simulink model "MCU_regionalPolePlacementLMI_SAME54_MCLV2"  (R2023b)
settings: Solver=FixedStepDiscrete  StartTime=0.0  StopTime=10.0  FixedStep=5e-5  RelTol=1e-3  EnableMultiTasking=on
InitFcn:
  | % DC Voltage
  | VDC = 24;
  | 
  | % Intersective PMW
  | Vmax = VDC/2;
  | Imax = 4;
  | 
  | Ts = 1e-4;
  | 
  | % pole paires
  | p = 4;
  | 
  | % QEI
  | lines = 4*1000;
  | eleclines = lines/p;
  | inveleclines = 1/eleclines
  | gainQEIspeed = 2*pi/Ts/lines
  | 
  | model.R = 0.656;         % Ohm
  | model.L = 0.35e-3;       % H
  | model.Phif = 6.6e-3;     % Wb
  | model.p = 4;
  | model.F = 1.e-05;
  | model.J = 1e-05;
  | disp(model);
  | 
  | % State space representation of the motor model
  | 
  | A = [-model.R/model.L -model.p*model.Phif ; 3*model.p*model.Phif/(2*model.J) -model.F/model.J ];
  | B = [1/model.L;0];
  | C = [0 1];
  | n=size(A,1);
  | % Augmented model with integral action
  | 
  | n=size(A,1); mx=size(B,2);
  | 
  | warning('off')
  | A = [A zeros(n,1);-C 0] ;
  | Bu=[B;0];Bw=[eye(3)];Duz=[1];Cz=[0 0 0];
  | 
  | n= 3;
  | m = 1;
  | 
  | %%% LIST OF UKNOWNS (lambda is the first, always included)
  | Nunk=uint16(2);
  | nunk = 1;
  | %UNK=cell(Nunk,1);
  | UNK = struct(...
  |     ...%'lab',{'X','Y'},...
  |     'col',{uint16(n),uint16(n)},...
  |     'row',{uint16(n),uint16(m)},...
  |     'sym',{uint16(1),uint16(0)},...
  |     'start',{uint16(0),uint16(0)},...
  |     'siz',{uint16(n*(n+1)/2),uint16(n*m)},...
  |     'X',{single(zeros(n,n,n*(n+1)/2)),single(zeros(m,n,n*m))},...
  |     'ste',{single(zeros(n,n)),single(zeros(m,n))},...
  |     'end',{uint16(nunk),uint16(nunk)}...
  |    );
  | 
  | 
  | ... (+100 lines)
undefined symbols (not defined in the file or in its folder): ADC0, AIN0, AIN6, B27, DiscIntNeverNeededParam, NumBits1, NumBits2, PA02, PA03, PA06, PA08, PA09, PA10, PA11, PA12, PA13, PA16, PA17, PA18, pad0, pad1, pad2, pad3, PB08, PC16, PC17, PC18, Pin, SAME54P20A, TQFP128, VREFA, wo0, wo1, wo2, wo4, wo5, wo6
libraries: simulink x20, MCHP_Blockset x12, dspfdesign x1
(part 2 of 3)

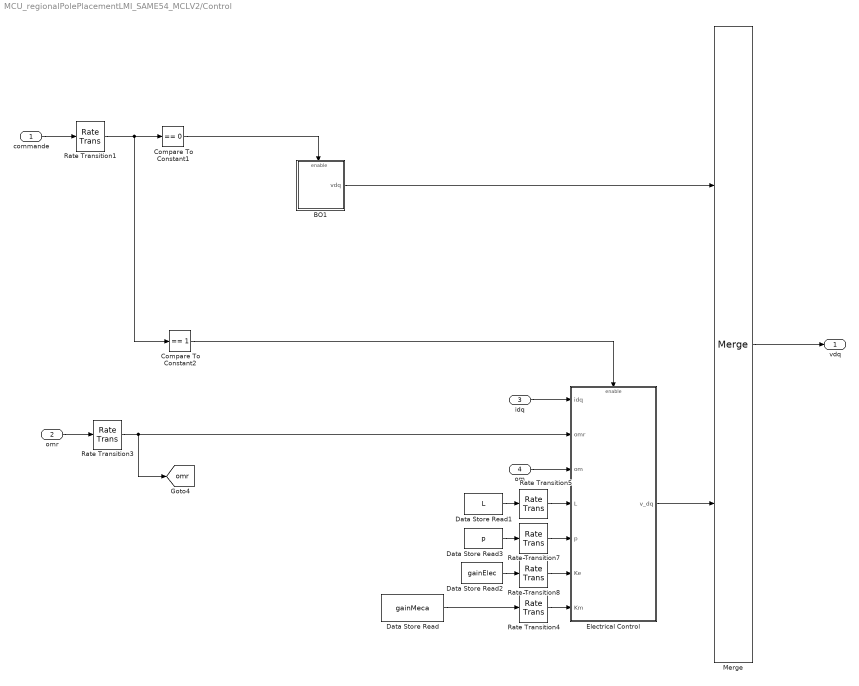
== system MCU_regionalPolePlacementLMI_SAME54_MCLV2/Control ==
  commande : Inport
  omr : Inport  Port=2
  idq : Inport  Port=3
  om : Inport  Port=4
  BO1 : Subsystem
  Compare To Constant1 : simulink/Logic and Bit Operations/Compare To Constant  relop===  const=0  OutDataTypeStr=boolean
  Compare To Constant2 : simulink/Logic and Bit Operations/Compare To Constant  relop===  const=1  OutDataTypeStr=boolean
  Data Store Read : DataStoreRead  DataStoreName=gainMeca  IndexOptions=Index vector (dialog)  Indices=1  OutputSizes=1
  Data Store Read1 : DataStoreRead  DataStoreName=L  SampleTime=1  IndexOptions=Index vector (dialog)  Indices=1  OutputSizes=1
  Data Store Read2 : DataStoreRead  DataStoreName=gainElec  IndexOptions=Index vector (dialog)  Indices=1  OutputSizes=1
  Data Store Read3 : DataStoreRead  DataStoreName=p  SampleTime=1  IndexOptions=Index vector (dialog)  Indices=1  OutputSizes=1
  Electrical Control : Subsystem
  Merge : Merge
  Rate Transition{1,3..5,7..8} (6 alike) : RateTransition
  vdq : Outport  VectorParamsAs1DForOutWhenUnconnected=off
  tag scope: omr=global
  wires:
  idq/1 -> Electrical Control/1(idq)
  Rate Transition1/1 -> Compare To Constant1/1, Compare To Constant2/1
  Compare To Constant1/1 -> BO1/Enable
  commande/1 -> Rate Transition1/1
  Merge/1 -> vdq/1
  Compare To Constant2/1 -> Electrical Control/Enable
  BO1/1(vdq) -> Merge/1
  Rate Transition3/1 -> [omr], Electrical Control/2(omr)
  Data Store Read3/1 -> Rate Transition7/1
  Data Store Read1/1 -> Rate Transition5/1
  Data Store Read2/1 -> Rate Transition8/1
  Electrical Control/1(v_dq) -> Merge/2
  Rate Transition5/1 -> Electrical Control/4(L)
  Rate Transition7/1 -> Electrical Control/5(p)
  Rate Transition8/1 -> Electrical Control/6(Ke)
  om/1 -> Electrical Control/3(om)
  omr/1 -> Rate Transition3/1
  Data Store Read/1 -> Rate Transition4/1
  Rate Transition4/1 -> Electrical Control/7(Km)

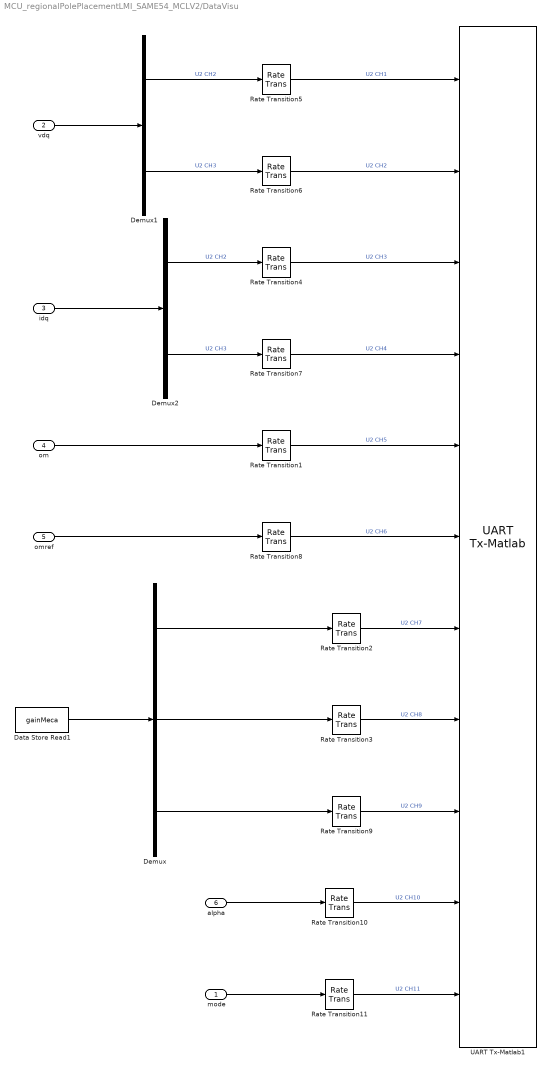
== system MCU_regionalPolePlacementLMI_SAME54_MCLV2/DataVisu ==
  mode : Inport
  vdq : Inport  Port=2
  idq : Inport  Port=3
  om : Inport  Port=4
  omref : Inport  Port=5
  alpha : Inport  Port=6
  Data Store Read1 : DataStoreRead  DataStoreName=gainMeca  IndexOptions=Index vector (dialog)  Indices=1  OutputSizes=1
  Demux : Demux  Outputs=3
  Demux1 : Demux  Outputs=2
  Demux2 : Demux  Outputs=2
  Rate Transition{1..9} (9 alike) : RateTransition
  Rate Transition10 : RateTransition  Integrity=off
  Rate Transition11 : RateTransition  Integrity=off
  UART Tx-Matlab1 : MCHP_Blockset/BUS UART/UART Tx-Matlab  UART_REF=2  CHANNELS=[1:11]  AllOrNothing=off  SampleTime=0.001  MCHP_MASTERLINK=MCU_regionalPolePlacementLMI_SAME54_MCLV2/Microchip Master  MCHP_COMPILED_INFO="CompiledSampleTime= [0.0010000000000000000208   0 ];CompiledInportDataTypes=[  1   1   1   1   1   1   1   1   1   1   5 ];CompiledInportDataWidth=[1  1  1  1  1  1  1  1  1  1  1];"
      settings: SourceProductName=MPLAB Device Blocks for Simulink
  wires:
  vdq/1 -> Demux1/1
  idq/1 -> Demux2/1
  omref/1 -> Rate Transition8/1
  Demux2/2 -> Rate Transition7/1  "U2 CH3"
  Demux2/1 -> Rate Transition4/1  "U2 CH2"
  Rate Transition5/1 -> UART Tx-Matlab1/1  "U2 CH1"
  Rate Transition8/1 -> UART Tx-Matlab1/6  "U2 CH6"
  Rate Transition1/1 -> UART Tx-Matlab1/5  "U2 CH5"
  Demux1/2 -> Rate Transition6/1  "U2 CH3"
  Rate Transition6/1 -> UART Tx-Matlab1/2  "U2 CH2"
  Rate Transition4/1 -> UART Tx-Matlab1/3  "U2 CH3"
  Demux1/1 -> Rate Transition5/1  "U2 CH2"
  om/1 -> Rate Transition1/1
  Rate Transition7/1 -> UART Tx-Matlab1/4  "U2 CH4"
  Rate Transition2/1 -> UART Tx-Matlab1/7  "U2 CH7"
  Rate Transition3/1 -> UART Tx-Matlab1/8  "U2 CH8"
  Rate Transition9/1 -> UART Tx-Matlab1/9  "U2 CH9"
  Demux/1 -> Rate Transition2/1
  Demux/2 -> Rate Transition3/1
  Demux/3 -> Rate Transition9/1
  Data Store Read1/1 -> Demux/1
  Rate Transition10/1 -> UART Tx-Matlab1/10  "U2 CH10"
  alpha/1 -> Rate Transition10/1
  mode/1 -> Rate Transition11/1
  Rate Transition11/1 -> UART Tx-Matlab1/11  "U2 CH11"

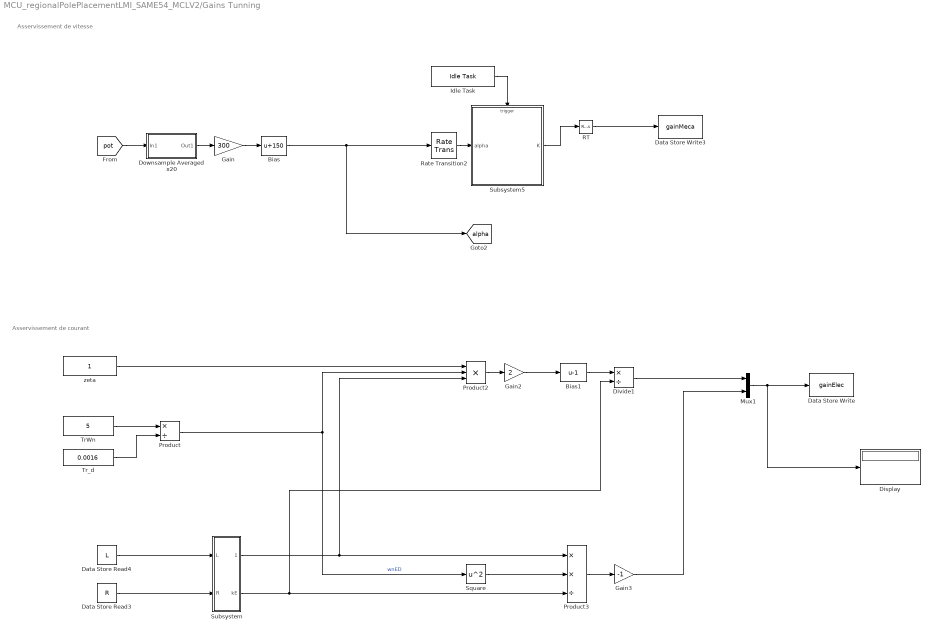
== system MCU_regionalPolePlacementLMI_SAME54_MCLV2/Gains Tunning ==
  note: Asservissement de courant
  note: Asservissement de vitesse
  Bias : Bias  Bias=150  SaturateOnIntegerOverflow=off
  Bias1 : Bias  Bias=-1  SaturateOnIntegerOverflow=off
  Data Store Read3 : DataStoreRead  DataStoreName=R  SampleTime=1  IndexOptions=Index vector (dialog)  Indices=1  OutputSizes=1
  Data Store Read4 : DataStoreRead  DataStoreName=L  SampleTime=1  IndexOptions=Index vector (dialog)  Indices=1  OutputSizes=1
  Data Store Write : DataStoreWrite  DataStoreName=gainElec  SampleTime=1  IndexOptions=Index vector (dialog)  Indices=1  OutputSizes=1
  Data Store Write3 : DataStoreWrite  DataStoreName=gainMeca  IndexOptions=Index vector (dialog)  Indices=1  OutputSizes=1
  Display : Display
  Divide1 : Product  Inputs=*/
  Downsample Averaged x20 : Subsystem  mask{DownSample=100}
      mask prompts: DownSample "DownSample Factor"
  Gain : Gain  Gain=300  OutDataTypeStr=single
  Gain2 : Gain  Gain=2
  Gain3 : Gain  Gain=-1
  Idle Task : MCHP_Blockset/System Functions/Idle Task  MCHP_MASTERLINK=MCU_regionalPolePlacementLMI_SAME54_MCLV2/Microchip Master
      settings: SourceProductName=MPLAB Device Blocks for Simulink
  Mux1 : Mux  Inputs=2
  Product : Product  Inputs=*/
  Product2 : Product  Inputs=3
  Product3 : Product  Inputs=**/
  RT : RateTransition  Deterministic=off  OutPortSampleTime=0.1
  Rate Transition2 : RateTransition  Integrity=off
  Square : Math  Operator=square
  Subsystem : Subsystem
  Subsystem5 : Subsystem
  TrWn : Constant  Value=5  OutDataTypeStr=single
  Tr_d : Constant  Value=0.0016  OutDataTypeStr=single
  zeta : Constant  OutDataTypeStr=single
  tag scope: alpha=global
  wires:
  Gain3/1 -> Mux1/2
  Product3/1 -> Gain3/1
  Divide1/1 -> Mux1/1
  Bias1/1 -> Divide1/1
  Product2/1 -> Gain2/1
  Mux1/1 -> Display/1, Data Store Write/1
  Data Store Read4/1 -> Subsystem/1(L)
  Data Store Read3/1 -> Subsystem/2(R)
  Subsystem/1(tauE) -> Product2/3, Product3/1
  TrWn/1 -> Product/1
  Tr_d/1 -> Product/2
  Product/1 -> Product2/2, Square/1  "wnED"
  Subsystem/2(kE) -> Divide1/2, Product3/3
  Gain2/1 -> Bias1/1
  zeta/1 -> Product2/1
  Square/1 -> Product3/2
  Downsample Averaged x20/1(Out1) -> Gain/1
  Gain/1 -> Bias/1
  Idle Task/1 -> Subsystem5/Trigger
  Rate Transition2/1 -> Subsystem5/1(alpha)
  Subsystem5/1(K) -> RT/1
  RT/1 -> Data Store Write3/1
  [pot] -> Downsample Averaged x20/1(In1)
  Bias/1 -> Rate Transition2/1, [alpha]

== system MCU_regionalPolePlacementLMI_SAME54_MCLV2/Inv Park ==
  cossin : Inport
  vdq : Inport  Port=2  PortDimensions=2
  Clakeinv : Subsystem
  ParkInv : Subsystem
  vabc : Outport  VectorParamsAs1DForOutWhenUnconnected=off
  wires:
  vdq/1 -> ParkInv/2(vdq)
  cossin/1 -> ParkInv/1(cos(pth)sin(pth))
  ParkInv/1(valbe) -> Clakeinv/1(alphabeta)
  Clakeinv/1(abc) -> vabc/1

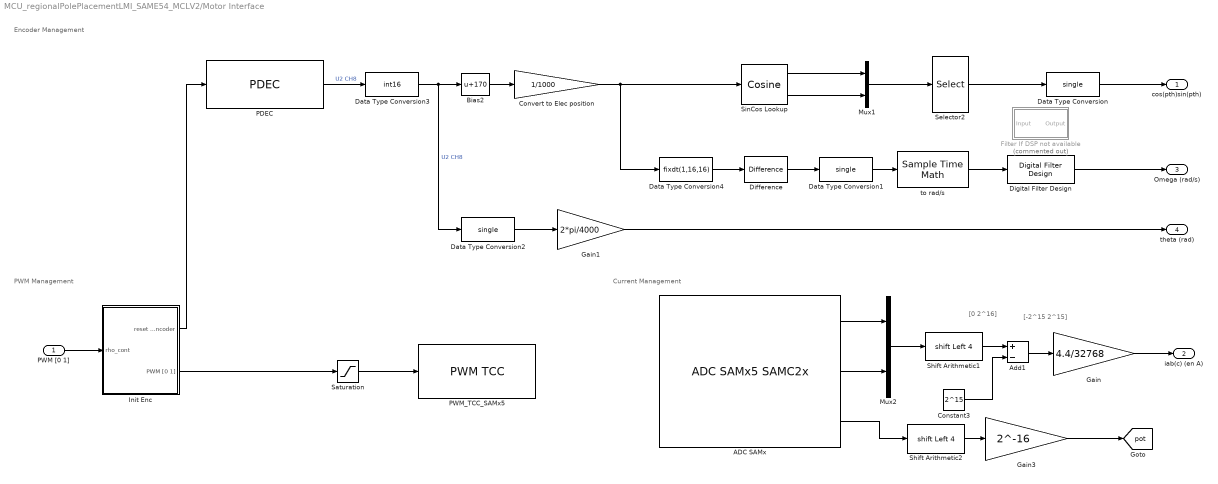
== system MCU_regionalPolePlacementLMI_SAME54_MCLV2/Motor Interface ==
  note: Encoder Management
  note: PWM Management
  note: [0 2^16]
  note: [-2^15 2^15]
  note: Current Management
  PWM [0 1] : Inport
  ADC SAMx : MCHP_Blockset/Analog IO/ADC SAMx5 SAMC2x  ADCREF=ADC 0 and ADC 1 (slave)  VREF_seq0=Dynamic Options  VREF_seq0_TXT=PA03 / VREFA / Pin[10]  info=0  SampleTime=1e-4  MCHP_PORT={ADC0_seq0.0}{ADC0_AIN0}15:2:P2;{ADC0_seq1.0}{ADC0_AIN6}15:2:P6;{ADC1_seq0.0}{ADC1_AIN0}15:2:P40;  MCHP_MASTERLINK=MCU_regionalPolePlacementLMI_SAME54_MCLV2/Microchip Master  MCHP_CRC=4646605  TrigSource_seq0=Dynamic Options  TrigSource_seq0_TXT=TCC0 PWM event Overflow - Period  ADC0_seq0=Dynamic Options  ADC0_seq0_TXT=PA02 / AIN0 / Pin[9]  ADC1_seq0=Dynamic Options  ADC1_seq0_TXT=PB08 / AIN0 / Pin[19]  ADC0_seq0_1=Dynamic Options  ADC0_seq0_1_TXT=Not Used  ADC1_seq0_1=Dynamic Options  ADC1_seq0_1_TXT=Not Used  ADC0_seq0_2=Dynamic Options  ADC0_seq0_2_TXT=Not Used  ADC1_seq0_2=Dynamic Options  ADC1_seq0_2_TXT=Not Used  ADC0_seq0_3=Dynamic Options  ADC0_seq0_3_TXT=Not Used  ADC1_seq0_3=Dynamic Options  ADC1_seq0_3_TXT=Not Used  ADC0_seq0_4=Dynamic Options  ADC0_seq0_4_TXT=Not Used  ADC1_seq0_4=Dynamic Options  ADC1_seq0_4_TXT=Not Used  ADC0_seq0_5=Dynamic Options  ADC0_seq0_5_TXT=Not Used  ADC1_seq0_5=Dynamic Options  ADC1_seq0_5_TXT=Not Used  Resolution_seq0=12 bits  SampleTime_seq0_s=1e-6  TrigTimeStep_seq0=on  info_seq0=0  TrigSource_seq1=Dynamic Options  TrigSource_seq1_TXT=after previous sequence  ADC0_seq1=Dynamic Options  ADC0_seq1_TXT=PA06 / AIN6 / Pin[23]  ADC1_seq1=Dynamic Options  ADC1_seq1_TXT=Not Used  ADC0_seq1_1=Dynamic Options  ADC0_seq1_1_TXT=Not Used  ADC1_seq1_1=Dynamic Options  ADC1_seq1_1_TXT=Not Used  ADC0_seq1_2=Dynamic Options  ADC0_seq1_2_TXT=Not Used  ADC1_seq1_2=Dynamic Options  ADC1_seq1_2_TXT=Not Used  ADC0_seq1_3=Dynamic Options  ADC0_seq1_3_TXT=Not Used  ADC1_seq1_3=Dynamic Options  ADC1_seq1_3_TXT=Not Used  ADC0_seq1_4=Dynamic Options  ADC0_seq1_4_TXT=Not Used  ADC1_seq1_4=Dynamic Options  ADC1_seq1_4_TXT=Not Used  ADC0_seq1_5=Dynamic Options  ADC0_seq1_5_TXT=Not Used  ADC1_seq1_5=Dynamic Options  ADC1_seq1_5_TXT=Not Used  Resolution_seq1=12 bits  SampleTime_seq1_s=1e-6  TrigTimeStep_seq1=off  info_seq1=0  TrigSource_seq2=Dynamic Options  TrigSource_seq2_TXT=after previous sequence  ADC0_seq2=Dynamic Options  ADC0_seq2_TXT=Not Used  ADC1_seq2=Dynamic Options  ADC1_seq2_TXT=Not Used  ADC0_seq2_1=Dynamic Options  ADC0_seq2_1_TXT=Not Used  ADC1_seq2_1=Dynamic Options  ADC1_seq2_1_TXT=Not Used  ADC0_seq2_2=Dynamic Options  ADC0_seq2_2_TXT=Not Used  ADC1_seq2_2=Dynamic Options  ADC1_seq2_2_TXT=Not Used  ADC0_seq2_3=Dynamic Options  ADC0_seq2_3_TXT=Not Used  ADC1_seq2_3=Dynamic Options  ADC1_seq2_3_TXT=Not Used  ADC0_seq2_4=Dynamic Options  ADC0_seq2_4_TXT=Not Used  ADC1_seq2_4=Dynamic Options  ADC1_seq2_4_TXT=Not Used  ADC0_seq2_5=Dynamic Options  ADC0_seq2_5_TXT=Not Used  ADC1_seq2_5=Dynamic Options  ADC1_seq2_5_TXT=Not Used  Resolution_seq2=12 bits  SampleTime_seq2_s=1e-6  TrigTimeStep_seq2=off  info_seq2=0  TrigSource_seq3=Dynamic Options  TrigSource_seq3_TXT=after previous sequence  ADC0_seq3=Dynamic Options  ADC0_seq3_TXT=Not Used  ADC1_seq3=Dynamic Options  ADC1_seq3_TXT=Not Used  ADC0_seq3_1=Dynamic Options  ADC0_seq3_1_TXT=Not Used  ADC1_seq3_1=Dynamic Options  ADC1_seq3_1_TXT=Not Used  ADC0_seq3_2=Dynamic Options  ADC0_seq3_2_TXT=Not Used  ADC1_seq3_2=Dynamic Options  ADC1_seq3_2_TXT=Not Used  ADC0_seq3_3=Dynamic Options  ADC0_seq3_3_TXT=Not Used  ADC1_seq3_3=Dynamic Options  ADC1_seq3_3_TXT=Not Used  ADC0_seq3_4=Dynamic Options  ADC0_seq3_4_TXT=Not Used  ADC1_seq3_4=Dynamic Options  ADC1_seq3_4_TXT=Not Used  ADC0_seq3_5=Dynamic Options  ADC0_seq3_5_TXT=Not Used  ADC1_seq3_5=Dynamic Options  ADC1_seq3_5_TXT=Not Used  Resolution_seq3=12 bits  SampleTime_seq3_s=1e-6  TrigTimeStep_seq3=off  info_seq3=0  TrigSource_seq4=Dynamic Options  TrigSource_seq4_TXT=after previous sequence  ADC0_seq4=Dynamic Options  ADC0_seq4_TXT=Not Used  ADC1_seq4=Dynamic Options  ADC1_seq4_TXT=Not Used  ADC0_seq4_1=Dynamic Options  ADC0_seq4_1_TXT=Not Used  ADC1_seq4_1=Dynamic Options  ADC1_seq4_1_TXT=Not Used  ADC0_seq4_2=Dynamic Options  ADC0_seq4_2_TXT=Not Used  ADC1_seq4_2=Dynamic Options  ADC1_seq4_2_TXT=Not Used  ADC0_seq4_3=Dynamic Options  ADC0_seq4_3_TXT=Not Used  ADC1_seq4_3=Dynamic Options  ADC1_seq4_3_TXT=Not Used  ADC0_seq4_4=Dynamic Options  ADC0_seq4_4_TXT=Not Used  ADC1_seq4_4=Dynamic Options  ADC1_seq4_4_TXT=Not Used  ADC0_seq4_5=Dynamic Options  ADC0_seq4_5_TXT=Not Used  ADC1_seq4_5=Dynamic Options  ADC1_seq4_5_TXT=Not Used  Resolution_seq4=12 bits  SampleTime_seq4_s=1e-6  TrigTimeStep_seq4=off  info_seq4=0  TrigSource_seq5=Dynamic Options  TrigSource_seq5_TXT=after previous sequence  ADC0_seq5=Dynamic Options  ADC0_seq5_TXT=Not Used  ADC1_seq5=Dynamic Options  ADC1_seq5_TXT=Not Used  ADC0_seq5_1=Dynamic Options  ADC0_seq5_1_TXT=Not Used  ADC1_seq5_1=Dynamic Options  ADC1_seq5_1_TXT=Not Used  ADC0_seq5_2=Dynamic Options  ADC0_seq5_2_TXT=Not Used  ADC1_seq5_2=Dynamic Options  ADC1_seq5_2_TXT=Not Used  ADC0_seq5_3=Dynamic Options  ADC0_seq5_3_TXT=Not Used  ADC1_seq5_3=Dynamic Options  ADC1_seq5_3_TXT=Not Used  ADC0_seq5_4=Dynamic Options  ADC0_seq5_4_TXT=Not Used  ADC1_seq5_4=Dynamic Options  ADC1_seq5_4_TXT=Not Used  ADC0_seq5_5=Dynamic Options  ADC0_seq5_5_TXT=Not Used  ADC1_seq5_5=Dynamic Options  ADC1_seq5_5_TXT=Not Used  Resolution_seq5=12 bits  SampleTime_seq5_s=1e-6  TrigTimeStep_seq5=off  info_seq5=0
      settings: SourceProductName=MPLAB Device Blocks for Simulink
  Add1 : Sum  Inputs=+-  OutDataTypeStr=single
  Bias2 : Bias  Bias=170  SaturateOnIntegerOverflow=off
  Constant3 : Constant  Value=2^15  OutDataTypeStr=fixdt(0,16,0)
  Convert to Elec position : Gain  Gain=1/1000  OutDataTypeStr=fixdt(0,16,16)
  Data Type Conversion : DataTypeConversion  OutDataTypeStr=single  SaturateOnIntegerOverflow=off  RndMeth=Floor
  Data Type Conversion1 : DataTypeConversion  OutDataTypeStr=single  SaturateOnIntegerOverflow=off  RndMeth=Floor
  Data Type Conversion2 : DataTypeConversion  OutDataTypeStr=single  SaturateOnIntegerOverflow=off  RndMeth=Floor
  Data Type Conversion3 : DataTypeConversion  OutDataTypeStr=int16  ConvertRealWorld=Stored Integer (SI)  SaturateOnIntegerOverflow=off  RndMeth=Floor
  Data Type Conversion4 : DataTypeConversion  OutDataTypeStr=fixdt(1,16,16)  ConvertRealWorld=Stored Integer (SI)  SaturateOnIntegerOverflow=off  RndMeth=Floor
  Difference : simulink/Discrete/Difference  ICPrevInput=0  OutMin=[]  OutMax=[]  OutDataType=fixdt(1, 16)  OutScaling=2^-10  DoSatur=off
  Digital Filter Design : dspfdesign/Digital Filter Design  mwdsp_browser_bugfix_var=off
  Filter If DSP not available : Subsystem  Tag=FilterWizardSubSystem  Commented=on
      settings: ErrorFcn=dspFilterRealizedInBasicElemsAlgLoopErrFcnCallback
  Gain : Gain  Gain=4.4/32768
  Gain1 : Gain  Gain=2*pi/4000
  Gain3 : Gain  Gain=2^-16  OutDataTypeStr=single
  Init Enc : Subsystem
  Mux1 : Mux  Inputs=2
  Mux2 : Mux  Inputs=2
  PDEC : MCHP_Blockset/QEI/PDEC  Mode=Quadrature Encoder  index=Reset counter  QDI0=PC16 / Pin[70]  QDI0_txt=Dynamic Options  QDI1=PC17 / Pin[71]  QDI1_txt=Dynamic Options  QDI2=PC18 / Pin[72]  QDI2_txt=Dynamic Options  maxCounterReset=-1  AutoCorrection=off  AutoCorrection_override=on  info=0  MCHP_MASTERLINK=MCU_regionalPolePlacementLMI_SAME54_MCLV2/Microchip Master  SampleTime=1e-4  MCHP_PORT={PDEC A}{PDEC_QDI0}5:0:P80;{PDEC B}{PDEC_QDI1}5:0:P81;{PDEC index}{PDEC_QDI2}5:0:P82;  MAXPOS_INPUT=off  RESET_INPUT=on  OutputCounter=on  OutputCounter_Signed=unsigned  OutputRevolution=off  CounterRevolution_length=Counter is 13 bits ; revolution is 3 bits  OutputRevolution_Signed=unsigned  FILTER="250 (ns)  ->  freq 2 (MHz)"  FILTER_TXT="250 (ns)  ->  freq 2 (MHz)"  SWAP=off  QDI_invert_0=off  QDI_invert_1=off  QDI_invert_2=off
      settings: SourceProductName=MPLAB Device Blocks for Simulink
  PWM_TCC_SAMx5 : MCHP_Blockset/PWM IO/PWM TCC  TCCREF=TCC 0  WAVE_choice=Center aligned PWM  MaxPeriod_s=5e-5  OTMX=Default  WO0=Dynamic Options  WO0_TXT=PA08 / Pin[33] / wo0  WO1=Dynamic Options  WO1_TXT=PA09 / Pin[34] / wo1  WO2=Dynamic Options  WO2_TXT=PA10 / Pin[35] / wo2  WO3=Dynamic Options  WO3_TXT=Not Used  WO4=Dynamic Options  WO4_TXT=PA16 / Pin[66] / wo4  WO5=Dynamic Options  WO5_TXT=PA17 / Pin[67] / wo5  WO6=Dynamic Options  WO6_TXT=PA18 / Pin[68] / wo6  WO7=Dynamic Options  WO7_TXT=Not Used  info=0  evalin_ws=PWM0max=MCHP_Fun.Hex2num('40A3860000000000');PWM0max=MCHP_Fun.Hex2num('40A3860000000000');PWM0max=MCHP_Fun.Hex2num('40A3860000000000');  SampleTime=1e-4  MCHP_PORT={PWM0_H0}{TCC0_WO0}5:1:P8;{PWM0_H1}{TCC0_WO1}5:1:P9;{PWM0_H2}{TCC0_WO2}5:1:P10;{PWM0_L0}{TCC0_WO4}5:1:P16;{PWM0_L1}{TCC0_WO5}5:1:P17;{PWM0_L2}{TCC0_WO6}5:1:P18;  MCHP_MASTERLINK=MCU_regionalPolePlacementLMI_SAME54_MCLV2/Microchip Master  INVEN_WO0=off  INVEN_WO1=off  INVEN_WO2=off  INVEN_WO3=off  INVEN_WO4=off  INVEN_WO5=off  INVEN_WO6=off  INVEN_WO7=off  SWAP_PWM0=off  SWAP_PWM1=off  SWAP_PWM2=off  SWAP_PWM3=off  POL_PWM0=off  POL_PWM1=off  POL_PWM2=off  POL_PWM3=off  POL_PWM4=off  POL_PWM5=off  InitPeriod_s=5e-5  InitDutyCycle_s=2.5e-5  InitDeadTimeH_s=0.5e-6  InitDeadTimeL_s=0.5e-6  InitOutputOverride=0  InitOutputOverride_val=0  BlockInput_VectorScalar=Vectors (grouped by function)  BlockInput_Period=Not a block input  BlockInput_DutyCycle=a Floating Point input within range [0 1]  BlockInput_DeadTime=Not a block input  BlockInput_OutputOverride=Not a block input
      settings: SourceProductName=MPLAB Device Blocks for Simulink
  Saturation : Saturate  UpperLimit=0.98  LowerLimit=0.02  LinearizeAsGain=off  OutDataTypeStr=double
  Selector2 : Selector  InputPortWidth=2  IndexOptions=Index vector (dialog)  Indices=[2 1]  OutputSizes=1
  Shift Arithmetic1 : ArithShift  BitShiftNumber=4  BitShiftDirection=Left
  Shift Arithmetic2 : ArithShift  BitShiftNumber=4  BitShiftDirection=Left
  SinCos Lookup : simulink/Lookup Tables/Cosine  Formula=sin(2*pi*u) and cos(2*pi*u)  NumDataPoints=(2^12)+1  OutputWordLength=16  InternalRulePriority=Precision
  to rad/s : SampleTimeMath  TsampMathOp=/  weightValue=(4)/(2*pi)
  cos(pth)sin(pth) : Outport  VectorParamsAs1DForOutWhenUnconnected=off
  iab(c) (en A) : Outport  Port=2  VectorParamsAs1DForOutWhenUnconnected=off
  Omega (rad/s) : Outport  Port=3  PortDimensions=1  VectorParamsAs1DForOutWhenUnconnected=off
  theta (rad) : Outport  Port=4  VectorParamsAs1DForOutWhenUnconnected=off
  tag scope: pot=global
  wires:
  Saturation/1 -> PWM_TCC_SAMx5/1
  Init Enc/2(PWM [0 1]) -> Saturation/1
  Convert to Elec position/1 -> Data Type Conversion4/1, SinCos Lookup/1
  to rad/s/1 -> Digital Filter Design/1
  Bias2/1 -> Convert to Elec position/1
  PDEC/1 -> Data Type Conversion3/1  "U2 CH8"
  Digital Filter Design/1 -> Omega (rad/s)/1
  Data Type Conversion/1 -> cos(pth)sin(pth)/1
  Mux1/1 -> Selector2/1
  Selector2/1 -> Data Type Conversion/1
  SinCos Lookup/2 -> Mux1/2
  SinCos Lookup/1 -> Mux1/1
  Data Type Conversion3/1 -> Data Type Conversion2/1, Bias2/1  "U2 CH8"
  Data Type Conversion2/1 -> Gain1/1
  Gain1/1 -> theta (rad)/1
  Difference/1 -> Data Type Conversion1/1
  Data Type Conversion4/1 -> Difference/1
  Data Type Conversion1/1 -> to rad/s/1
  Shift Arithmetic2/1 -> Gain3/1
  Gain/1 -> iab(c) (en A)/1
  Gain3/1 -> [pot]
  Add1/1 -> Gain/1
  Mux2/1 -> Shift Arithmetic1/1
  Shift Arithmetic1/1 -> Add1/1
  ADC SAMx/2 -> Mux2/2
  Constant3/1 -> Add1/2
  ADC SAMx/1 -> Mux2/1
  ADC SAMx/3 -> Shift Arithmetic2/1
  Init Enc/1(reset encoder) -> PDEC/1
  PWM [0 1]/1 -> Init Enc/1(rho_cont)

== system MCU_regionalPolePlacementLMI_SAME54_MCLV2/PWM ==
  vabc : Inport
  50% average duty-cycle : Bias  Bias=0.5  SaturateOnIntegerOverflow=off
  Gain : Gain  Gain=1/VDC  OutDataTypeStr=double
  PWM [0 1] : Outport  VectorParamsAs1DForOutWhenUnconnected=off
  wires:
  vabc/1 -> Gain/1
  50% average duty-cycle/1 -> PWM [0 1]/1
  Gain/1 -> 50% average duty-cycle/1

== system MCU_regionalPolePlacementLMI_SAME54_MCLV2/Park  ==
  cossin : Inport
  xab(c) : Inport  Port=2
  Clark Fixe : Subsystem
  Park Fixe : Subsystem
  xdq : Outport  VectorParamsAs1DForOutWhenUnconnected=off
  wires:
  Clark Fixe/1(xalphabeta) -> Park Fixe/1(xalphabeta)
  xab(c)/1 -> Clark Fixe/1(xab(c))
  cossin/1 -> Park Fixe/2(cos(pth)sin(pth))
  Park Fixe/1(xdq) -> xdq/1

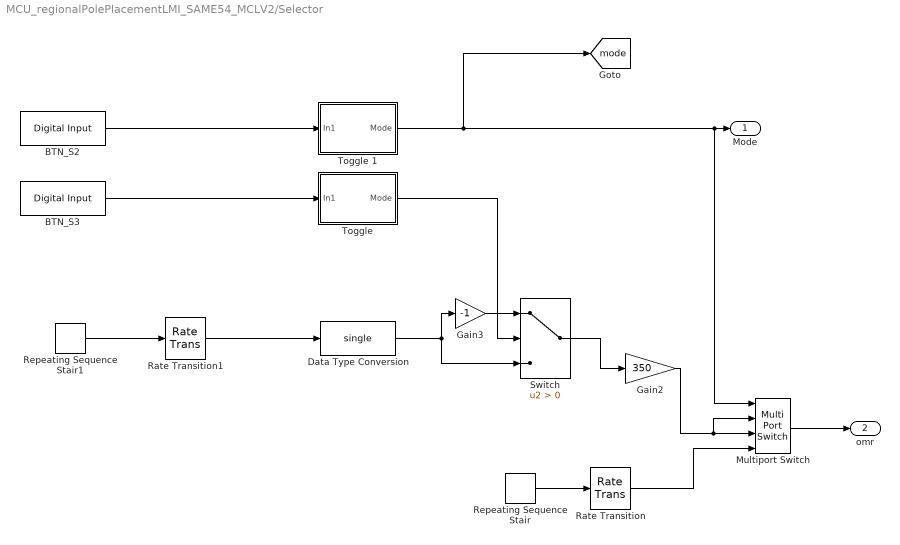
== system MCU_regionalPolePlacementLMI_SAME54_MCLV2/Selector ==
  BTN_S2 : MCHP_Blockset/Digital IO/Digital Input  PORT=Dynamic Options  PORT_TXT="D   [ 0  1  8  9  10  11  12  20  21 ]"  PIN=9  PACK=off  SIMULTANEOUS=off  ORDERING=None  SampleTime=.1  MCHP_PORT={Digital In}{DIN}2:0:D9;  MCHP_MASTERLINK=MCU_regionalPolePlacementLMI_SAME54_MCLV2/Microchip Master
      settings: SourceProductName=MPLAB Device Blocks for Simulink
  BTN_S3 : MCHP_Blockset/Digital IO/Digital Input  PORT=Dynamic Options  PORT_TXT="D   [ 0  1  8  9  10  11  12  20  21 ]"  PIN=10  PACK=off  SIMULTANEOUS=off  ORDERING=None  SampleTime=.1  MCHP_PORT={Digital In}{DIN}2:0:D10;  MCHP_MASTERLINK=MCU_regionalPolePlacementLMI_SAME54_MCLV2/Microchip Master
      settings: SourceProductName=MPLAB Device Blocks for Simulink
  Data Type Conversion : DataTypeConversion  OutDataTypeStr=single  SaturateOnIntegerOverflow=off  RndMeth=Floor
  Gain2 : Gain  Gain=350
  Gain3 : Gain  Gain=-1
  Multiport Switch : MultiPortSwitch  DataPortIndices={2,3}  SaturateOnIntegerOverflow=off  InputSameDT=off
  Rate Transition : RateTransition
  Rate Transition1 : RateTransition  OutPortSampleTime=0.1
  Repeating Sequence Stair : simulink/Sources/Repeating Sequence Stair  OutValues=[100 200].'  tsamp=1  OutMin=[]  OutMax=[]  OutDataTypeStr=single  OutputDataTypeScalingMode=single  OutDataType=fixdt(0,8)  ConRadixGroup=Best Precision: Vector-wise  OutScaling=2^-12
  Repeating Sequence Stair1 : simulink/Sources/Repeating Sequence Stair  OutValues=[100/350 200/350].'  tsamp=1  OutMin=[]  OutMax=[]  OutDataTypeStr=double  OutputDataTypeScalingMode=double  OutDataType=fixdt(0,8)  ConRadixGroup=Best Precision: Vector-wise  OutScaling=2^-12
  Switch : Switch  Criteria=u2 > Threshold  SaturateOnIntegerOverflow=off  InputSameDT=off
  Toggle : Subsystem
  Toggle 1 : Subsystem
  Mode : Outport  VectorParamsAs1DForOutWhenUnconnected=off
  omr : Outport  Port=2  VectorParamsAs1DForOutWhenUnconnected=off
  tag scope: mode=global
  wires:
  BTN_S2/1 -> Toggle 1/1(In1)
  Gain2/1 -> Multiport Switch/2, Multiport Switch/3
  Switch/1 -> Gain2/1
  Toggle 1/1(Mode) -> [mode], Multiport Switch/1, Mode/1
  Repeating Sequence Stair1/1 -> Rate Transition1/1
  Rate Transition1/1 -> Data Type Conversion/1
  BTN_S3/1 -> Toggle/1(In1)
  Toggle/1(Mode) -> Switch/2
  Data Type Conversion/1 -> Gain3/1, Switch/3
  Gain3/1 -> Switch/1
  Repeating Sequence Stair/1 -> Rate Transition/1
  Multiport Switch/1 -> omr/1
  Rate Transition/1 -> Multiport Switch/4

== system MCU_regionalPolePlacementLMI_SAME54_MCLV2/Control/BO1 ==
  Enable : EnablePort
  Mux : Mux  Inputs=2
  vd : Constant  Value=0  OutMin=[-12]  OutMax=[12]  OutDataTypeStr=single
  vq : Constant  Value=0  OutMin=[-12]  OutMax=[12]  OutDataTypeStr=single
  vdq : Outport  VectorParamsAs1DForOutWhenUnconnected=off
  wires:
  vd/1 -> Mux/1
  Mux/1 -> vdq/1
  vq/1 -> Mux/2

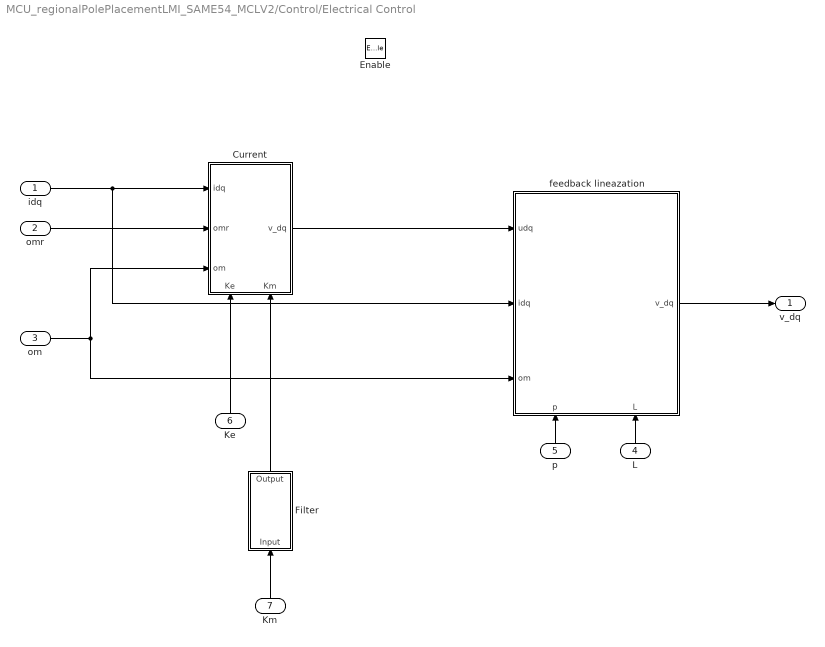
== system MCU_regionalPolePlacementLMI_SAME54_MCLV2/Control/Electrical Control ==
  idq : Inport
  omr : Inport  Port=2
  om : Inport  Port=3
  L : Inport  Port=4
  p : Inport  Port=5
  Ke : Inport  Port=6
  Km : Inport  Port=7
  Enable : EnablePort  StatesWhenEnabling=reset
  Current : Subsystem
      settings: PortSchema="{\"entries\":[{\"content\":{\"sides\":[{\"content\":{\"connectorIds\":[\"In1\",\"In2\",\"In3\"]},\"type\":\"ConnectorPlacement.EquallySpacedRectSide\",\"uuid\":\"0dd1bd5c-4f2d-4a51-9bc2-8bf74640d4ff\"},{\"content\":{\"connectorIds\":[\"Out1\"],\"side\":\"RIGHT\"},\"type\":\"ConnectorPlacement.EquallySpacedRectSide\",\"uuid\":\"9ff54608-efe8-47a2-97c0-1c2807ae0451\"},{\"content\":{\"connectorIds\":[],\"side\":\"TOP\"},\"type\":\"ConnectorPlacement.EquallySpacedRectSide\",\"uuid\":\"a5b0a1bc-2629-443b-a6ad-4c332df72e2c\"},{\"content\":{\"connectorIds\":[\"In4\",\"In5\"],\"side\":\"BOTTOM\"},\"type\":\"ConnectorPlacement.EquallySpacedRectSide\",\"uuid\":\"e8d63822-9705-4716-821c-9412f2966827\"},{\"content\":{\"connectorIds\":[],\"side\":\"HIDDEN\"},\"type\":\"ConnectorPlacement.EquallySpacedRectSide\",\"uuid\":\"63401b5c-75e9-49e9-aa08-12658d9987d3\"}]},\"type\":\"ConnectorPlacement.EquallySpacedConnector\",\"uuid\":\"d3f45542-3ea7-483a-a2ee-6c72d9ae8820\"}],\"packageUris\":[\"http://schema.mathworks.com/mf0/Connector/R2020b\"],\"version\":\"1.0\"}"
  Filter : Subsystem  Tag=FilterWizardSubSystem
      settings: ErrorFcn=dspFilterRealizedInBasicElemsAlgLoopErrFcnCallback
  feedback lineazation : Subsystem
      settings: PortSchema="{\"entries\":[{\"content\":{\"sides\":[{\"content\":{\"connectorIds\":[\"In1\",\"In2\",\"In3\"]},\"type\":\"ConnectorPlacement.EquallySpacedRectSide\",\"uuid\":\"169b5321-ee7c-423e-8449-192a786c9798\"},{\"content\":{\"connectorIds\":[\"Out1\"],\"side\":\"RIGHT\"},\"type\":\"ConnectorPlacement.EquallySpacedRectSide\",\"uuid\":\"910fdd05-0903-4759-8f85-a6669ffcf15d\"},{\"content\":{\"connectorIds\":[],\"side\":\"TOP\"},\"type\":\"ConnectorPlacement.EquallySpacedRectSide\",\"uuid\":\"8e0cf6ac-18cd-4e02-9312-1598b8dbe459\"},{\"content\":{\"connectorIds\":[\"In4\",\"In5\"],\"side\":\"BOTTOM\"},\"type\":\"ConnectorPlacement.EquallySpacedRectSide\",\"uuid\":\"bf7c0436-036d-4f64-97d8-e9b131650054\"},{\"content\":{\"connectorIds\":[],\"side\":\"HIDDEN\"},\"type\":\"ConnectorPlacement.EquallySpacedRectSide\",\"uuid\":\"cd87405f-25ee-425b-a181-6989070156fa\"}]},\"type\":\"ConnectorPlacement.EquallySpacedConnector\",\"uuid\":\"912b1b6f-c896-42c8-9325-248c15d73689\"}],\"packageUris\":[\"http://schema.mathworks.com/mf0/Connector/R2020b\"],\"version\":\"1.0\"}"
  v_dq : Outport
  wires:
  Ke/1 -> Current/4(Ke)
  idq/1 -> Current/1(idq), feedback lineazation/2(idq)
  Current/1(v_dq) -> feedback lineazation/1(udq)
  omr/1 -> Current/2(omr)
  feedback lineazation/1(v_dq) -> v_dq/1
  p/1 -> feedback lineazation/4(p)
  L/1 -> feedback lineazation/5(L)
  om/1 -> feedback lineazation/3(om), Current/3(om)
  Filter/1(Output) -> Current/5(Km)
  Km/1 -> Filter/1(Input)

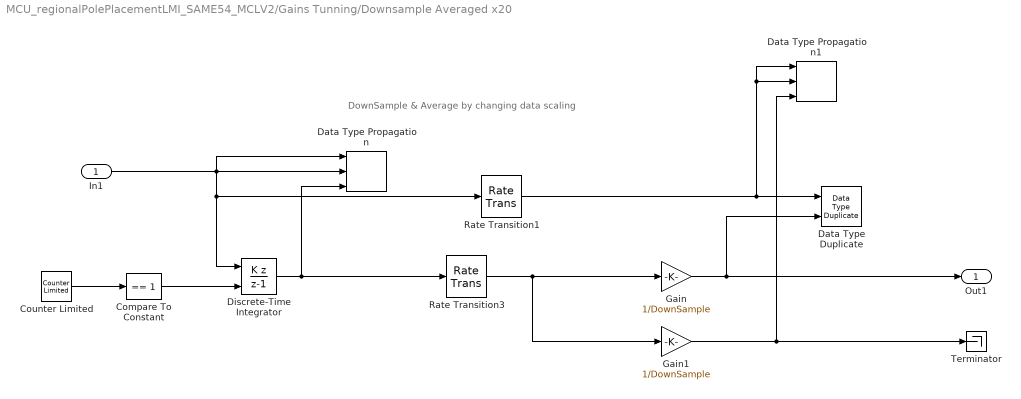
== system MCU_regionalPolePlacementLMI_SAME54_MCLV2/Gains Tunning/Downsample Averaged x20 ==
  note: DownSample & Average by changing data scaling
  In1 : Inport
  Compare To Constant : simulink/Logic and Bit Operations/Compare To Constant  relop===  const=1  OutDataTypeStr=boolean
  Counter Limited : simulink/Sources/Counter Limited  uplimit=DownSample-1  tsamp=-1
  Data Type Duplicate : DataTypeDuplicate
  Data Type Propagation : simulink/Signal Attributes/Data Type Propagation  PropDataType=fixdt(1, 16)  IfRefDouble=double  IfRefSingle=single  IsSigned=IsSigned1 or IsSigned2  NumBitsBase=NumBits1+NumBits2  NumBitsMult=1  NumBitsAdd=0  NumBitsAllowFinal=1:128  PropScaling=2^-10  ValuesUsedBestPrec=[5 -7]  SlopeBase=Slope1  SlopeMult=1  SlopeAdd=0  BiasBase=Bias1  BiasMult=1  BiasAdd=0
  Data Type Propagation1 : simulink/Signal Attributes/Data Type Propagation  PropDataType=fixdt(1, 16)  IfRefDouble=double  IfRefSingle=single  IsSigned=IsSigned1 or IsSigned2  NumBitsBase=NumBits1+NumBits2  NumBitsMult=1  NumBitsAdd=0  NumBitsAllowFinal=1:128  PropScaling=2^-10  ValuesUsedBestPrec=[5 -7]  SlopeBase=PosRange1  SlopeMult=1  SlopeAdd=0  BiasBase=Bias1  BiasMult=1  BiasAdd=0
  Discrete-Time Integrator : DiscreteIntegrator  IntegratorMethod=Accumulation: Backward Euler  gainval=1  ExternalReset=sampled level  SampleTime=-1  OutDataTypeStr=Inherit: Inherit via back propagation  ICPrevOutput=DiscIntNeverNeededParam  ICPrevScaledInput=DiscIntNeverNeededParam
  Gain : Gain  Gain=1/DownSample  OutDataTypeStr=Inherit: Inherit via back propagation  RndMeth=Round
  Gain1 : Gain  Gain=1/DownSample  OutDataTypeStr=Inherit: Inherit via back propagation
  Rate Transition1 : RateTransition  OutPortSampleTimeOpt=Multiple of input port sample time  OutPortSampleTimeMultiple=DownSample  OutPortSampleTime=DownSample
  Rate Transition3 : RateTransition  OutPortSampleTimeOpt=Multiple of input port sample time  OutPortSampleTimeMultiple=DownSample  OutPortSampleTime=DownSample
  Terminator : Terminator
  Out1 : Outport  VectorParamsAs1DForOutWhenUnconnected=off
  wires:
  Gain1/1 -> Data Type Propagation1/3, Terminator/1
  Rate Transition1/1 -> Data Type Duplicate/1, Data Type Propagation1/1, Data Type Propagation1/2
  Gain/1 -> Out1/1, Data Type Duplicate/2
  Counter Limited/1 -> Compare To Constant/1
  Discrete-Time Integrator/1 -> Rate Transition3/1, Data Type Propagation/3
  Compare To Constant/1 -> Discrete-Time Integrator/2
  In1/1 -> Data Type Propagation/1, Data Type Propagation/2, Discrete-Time Integrator/1, Rate Transition1/1
  Rate Transition3/1 -> Gain/1, Gain1/1

== system MCU_regionalPolePlacementLMI_SAME54_MCLV2/Gains Tunning/Subsystem ==
  L : Inport
  R : Inport  Port=2
  Divide1 : Product  Inputs=/
  Divide2 : Product  Inputs=*/
  tauE : Outport
  kE : Outport  Port=2
  wires:
  Divide2/1 -> tauE/1  "tauE"
  R/1 -> Divide1/1, Divide2/2
  L/1 -> Divide2/1
  Divide1/1 -> kE/1  "kE"

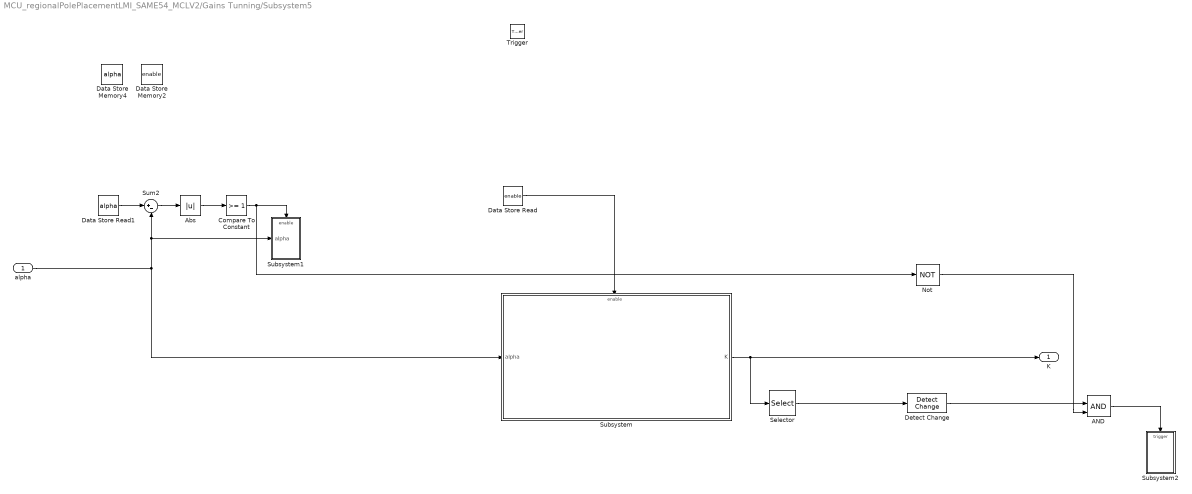
== system MCU_regionalPolePlacementLMI_SAME54_MCLV2/Gains Tunning/Subsystem5 ==
  alpha : Inport
  Trigger : TriggerPort  TriggerType=function-call  VariantControl=(inherit)  PortDimensions=1
  AND : Logic  IconShape=distinctive  AllPortsSameDT=off  OutDataTypeStr=boolean
  Abs : Abs  SaturateOnIntegerOverflow=off
  Compare To Constant : simulink/Logic and Bit Operations/Compare To Constant  relop=>=  const=1  OutDataTypeStr=boolean
  Data Store Memory2 : DataStoreMemory  DataStoreName=enable  ReadBeforeWriteMsg=warning  WriteAfterWriteMsg=warning  WriteAfterReadMsg=warning  ShowAdditionalParam=off  OutDataTypeStr=boolean
  Data Store Memory4 : DataStoreMemory  DataStoreName=alpha  ReadBeforeWriteMsg=warning  WriteAfterWriteMsg=warning  WriteAfterReadMsg=warning  ShowAdditionalParam=off  OutDataTypeStr=single
  Data Store Read : DataStoreRead  DataStoreName=enable  IndexOptions=Index vector (dialog)  Indices=1  OutputSizes=1
  Data Store Read1 : DataStoreRead  DataStoreName=alpha  IndexOptions=Index vector (dialog)  Indices=1  OutputSizes=1
  Detect Change : simulink/Logic and Bit Operations/Detect Change  vinit=0  OutDataTypeStr=boolean
      settings: LibrarySourceBlock=|
      | hdlsllib/Logic and Bit
      | Operations/Detect
      | Change
  Not : Logic  Operator=NOT  IconShape=distinctive  AllPortsSameDT=off  OutDataTypeStr=boolean
  Selector : Selector  InputPortWidth=3  IndexOptions=Index vector (dialog)  Indices=[3]  OutputSizes=1
  Subsystem : Subsystem
  Subsystem1 : Subsystem
  Subsystem2 : Subsystem
  Sum2 : Sum  Inputs=|+-
  K : Outport
  wires:
  AND/1 -> Subsystem2/Trigger
  Not/1 -> AND/2
  Data Store Read1/1 -> Sum2/1
  Selector/1 -> Detect Change/1
  Data Store Read/1 -> Subsystem/Enable
  Detect Change/1 -> AND/1
  Compare To Constant/1 -> Not/1, Subsystem1/Enable
  Abs/1 -> Compare To Constant/1
  Sum2/1 -> Abs/1
  Subsystem/1(K) -> Selector/1, K/1
  alpha/1 -> Subsystem/1(alpha), Subsystem1/1(alpha), Sum2/2

== system MCU_regionalPolePlacementLMI_SAME54_MCLV2/Inv Park/Clakeinv ==
  alphabeta : Inport
  Clarke1 : Product  Multiplication=Matrix(*)  RndMeth=Simplest  OutDataTypeStr=Inherit: Same as first input
  Constant Magnitude : Constant  Value=[1 0 ; -1/2 sqrt(3)/2 ;-1/2 -sqrt(3)/2]'  OutDataTypeStr=Inherit: Inherit via back propagation  SampleTime=-1
  Math Function : Math  Operator=transpose  SignedPower=on
  abc : Outport  VectorParamsAs1DForOutWhenUnconnected=off
  wires:
  alphabeta/1 -> Math Function/1
  Constant Magnitude/1 -> Clarke1/2
  Math Function/1 -> Clarke1/1
  Clarke1/1 -> abc/1

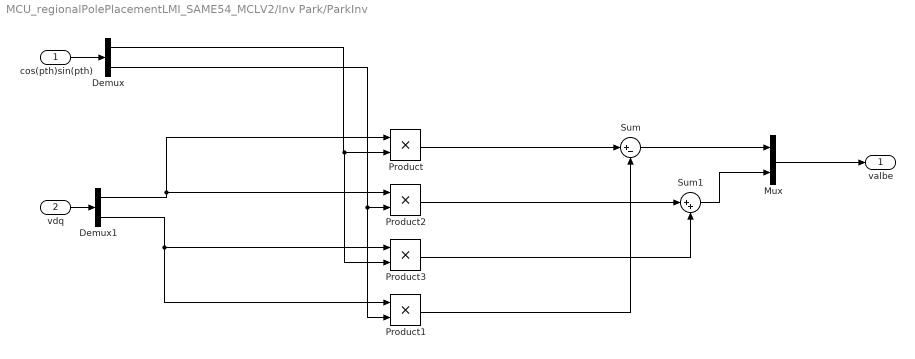
== system MCU_regionalPolePlacementLMI_SAME54_MCLV2/Inv Park/ParkInv ==
  cos(pth)sin(pth) : Inport
  vdq : Inport  Port=2
  Demux : Demux  Outputs=2
  Demux1 : Demux  Outputs=2
  Mux : Mux  Inputs=2
  Product{,1..3} (4 alike) : Product
  Sum : Sum  Inputs=|+-
  Sum1 : Sum  Inputs=|++
  valbe : Outport  VectorParamsAs1DForOutWhenUnconnected=off
  wires:
  vdq/1 -> Demux1/1
  cos(pth)sin(pth)/1 -> Demux/1
  Sum/1 -> Mux/1
  Demux1/1 -> Product2/1, Product/1
  Demux1/2 -> Product3/1, Product1/1
  Sum1/1 -> Mux/2
  Product1/1 -> Sum/2
  Product/1 -> Sum/1
  Demux/1 -> Product3/2, Product/2
  Demux/2 -> Product2/2, Product1/2
  Mux/1 -> valbe/1
  Product2/1 -> Sum1/1
  Product3/1 -> Sum1/2

== system MCU_regionalPolePlacementLMI_SAME54_MCLV2/Motor Interface/Filter If DSP not available ==
  Input : Inport
  Delay11 : Delay  DelayLength=1  InitialCondition=0
  Delay21 : Delay  DelayLength=1  InitialCondition=0
  SumA21 : Sum  Inputs=|+-  RndMeth=Nearest  SaturateOnIntegerOverflow=on  OutDataTypeStr=Inherit: Same as first input
  SumA31 : Sum  Inputs=|+-  RndMeth=Nearest  SaturateOnIntegerOverflow=on  OutDataTypeStr=Inherit: Same as first input
  SumB21 : Sum  Inputs=|++  RndMeth=Nearest  SaturateOnIntegerOverflow=on  OutDataTypeStr=Inherit: Same as first input
  SumB31 : Sum  Inputs=|++  RndMeth=Nearest  SaturateOnIntegerOverflow=on  OutDataTypeStr=Inherit: Same as first input
  a(2)(1) : Gain  Gain=-1.14298050253990113  ParamDataTypeStr=double  RndMeth=Nearest  SaturateOnIntegerOverflow=on  OutDataTypeStr=Inherit: Same as input
  a(3)(1) : Gain  Gain=0.412801598096188771  ParamDataTypeStr=double  RndMeth=Nearest  SaturateOnIntegerOverflow=on  OutDataTypeStr=Inherit: Same as input
  b(2)(1) : Gain  Gain=2  ParamDataTypeStr=double  RndMeth=Nearest  SaturateOnIntegerOverflow=on  OutDataTypeStr=Inherit: Same as input
  s(1) : Gain  Gain=0.0674552738890718956  ParamDataTypeStr=double  RndMeth=Nearest  SaturateOnIntegerOverflow=on  OutDataTypeStr=Inherit: Same as input
  Output : Outport
  wires:
  Delay21/1 -> SumB31/2, a(3)(1)/1
  a(3)(1)/1 -> SumA31/2
  b(2)(1)/1 -> SumB21/2
  Delay11/1 -> Delay21/1, b(2)(1)/1, a(2)(1)/1
  a(2)(1)/1 -> SumA21/2
  SumB31/1 -> Output/1
  SumB21/1 -> SumB31/1
  SumA31/1 -> Delay11/1, SumB21/1
  SumA21/1 -> SumA31/1
  s(1)/1 -> SumA21/1
  Input/1 -> s(1)/1

== system MCU_regionalPolePlacementLMI_SAME54_MCLV2/Motor Interface/Init Enc ==
  rho_cont : Inport
  Constant2 : Constant  Value=[.6 .5 .5]  OutDataTypeStr=Inherit: Inherit via back propagation
  Data Type Duplicate : DataTypeDuplicate
  Rate Transition1 : RateTransition
  Rate Transition2 : RateTransition
  Switch : Switch  Criteria=u2 > Threshold  SaturateOnIntegerOverflow=off  InputSameDT=off
  Wait 1s : Subsystem
  reset encoder : Outport
  PWM [0 1] : Outport  Port=2
  wires:
  Rate Transition2/1 -> Switch/2
  Rate Transition1/1 -> reset encoder/1
  Switch/1 -> PWM [0 1]/1, Data Type Duplicate/2
  Constant2/1 -> Switch/3
  Wait 1s/2(init done) -> Rate Transition2/1
  rho_cont/1 -> Switch/1, Data Type Duplicate/1
  Wait 1s/1(init enc) -> Rate Transition1/1

== system MCU_regionalPolePlacementLMI_SAME54_MCLV2/Park /Clark Fixe ==
  note: Input is a vector of 3 elements, 3rd element is not beeing used
  note: k = 2/3 : invariant Magnitude
  xab(c) : Inport
  Clarke1 : Product  Multiplication=Matrix(*)  OutDataTypeStr=single  RndMeth=Convergent  SaturateOnIntegerOverflow=on
  Constant Magnitude : Constant  Value=[1 0 ; 1/sqrt(3) 2/sqrt(3) ];  OutDataTypeStr=single
  xalphabeta : Outport  VectorParamsAs1DForOutWhenUnconnected=off
  wires:
  Clarke1/1 -> xalphabeta/1
  Constant Magnitude/1 -> Clarke1/1
  xab(c)/1 -> Clarke1/2

== system MCU_regionalPolePlacementLMI_SAME54_MCLV2/Park /Park Fixe ==
  xalphabeta : Inport
  cos(pth)sin(pth) : Inport  Port=2
  Demux : Demux  Outputs=2
  Demux1 : Demux  Outputs=2
  Mux : Mux  Inputs=2
  Product{,1..3} (4 alike) : Product
  Sum : Sum  Inputs=|++  SaturateOnIntegerOverflow=on
  Sum1 : Sum  Inputs=|-+  SaturateOnIntegerOverflow=on
  xdq : Outport  VectorParamsAs1DForOutWhenUnconnected=off
  wires:
  cos(pth)sin(pth)/1 -> Demux1/1
  Product2/1 -> Sum1/2
  Product1/1 -> Sum1/1
  Demux1/2 -> Product3/2, Product1/2
  Demux1/1 -> Product2/2, Product/2
  Product/1 -> Sum/1
  Product3/1 -> Sum/2
  Sum1/1 -> Mux/2
  Demux/2 -> Product3/1, Product2/1
  Demux/1 -> Product1/1, Product/1
  Sum/1 -> Mux/1
  Mux/1 -> xdq/1
  xalphabeta/1 -> Demux/1

== system MCU_regionalPolePlacementLMI_SAME54_MCLV2/Selector/Toggle ==
  In1 : Inport
  Bitwise Operator : simulink/Logic and Bit Operations/Bitwise Operator  logicop=AND  UseBitMask=on  BitMask=1  BitMaskRealWorld=Stored Integer
  Change when button is pressed : simulink/Logic and Bit Operations/Detect Decrease  vinit=0.0  OutDataTypeStr=uint8
  Sum : Sum  OutDataTypeStr=uint16  AccumDataTypeStr=uint16
  Unit Delay : UnitDelay  SampleTime=-1  HasFrameUpgradeWarning=on
  Mode : Outport  VectorParamsAs1DForOutWhenUnconnected=off
  wires:
  In1/1 -> Change when button is pressed/1
  Sum/1 -> Bitwise Operator/1
  Unit Delay/1 -> Sum/2
  Bitwise Operator/1 -> Unit Delay/1, Mode/1
  Change when button is pressed/1 -> Sum/1

== system MCU_regionalPolePlacementLMI_SAME54_MCLV2/Selector/Toggle 1 ==
  In1 : Inport
  Bitwise Operator : simulink/Logic and Bit Operations/Bitwise Operator  logicop=AND  UseBitMask=on  BitMask=1  BitMaskRealWorld=Stored Integer
  Change when button is pressed : simulink/Logic and Bit Operations/Detect Decrease  vinit=0.0  OutDataTypeStr=uint8
  Sum : Sum  OutDataTypeStr=uint16  AccumDataTypeStr=uint16
  Unit Delay : UnitDelay  SampleTime=-1  HasFrameUpgradeWarning=on
  Mode : Outport  VectorParamsAs1DForOutWhenUnconnected=off
  wires:
  Change when button is pressed/1 -> Sum/1
  Bitwise Operator/1 -> Mode/1, Unit Delay/1
  Unit Delay/1 -> Sum/2
  Sum/1 -> Bitwise Operator/1
  In1/1 -> Change when button is pressed/1

== system MCU_regionalPolePlacementLMI_SAME54_MCLV2/Control/Electrical Control/Current ==
  idq : Inport
  omr : Inport  Port=2
  om : Inport  Port=3
  Ke : Inport  Port=4
  Km : Inport  Port=5
  Constant : Constant  Value=0  OutDataTypeStr=single
  Gain1 : Gain  Gain=[1 0]  Multiplication=Matrix(K*u)  OutDataTypeStr=Inherit: Same as input
  Gain2 : Gain  Gain=[0 1]  Multiplication=Matrix(K*u)  OutDataTypeStr=Inherit: Same as input
  Mux1 : Mux  Inputs=2
  Subsystem1 : Subsystem
  Subsystem2 : Subsystem
  v_dq : Outport  VectorParamsAs1DForOutWhenUnconnected=off
  wires:
  om/1 -> Subsystem2/2(om)
  Gain2/1 -> Subsystem2/3(i)
  omr/1 -> Subsystem2/1(omref)
  Ke/1 -> Subsystem1/3(K_e)
  Mux1/1 -> v_dq/1
  Gain1/1 -> Subsystem1/2(i)
  idq/1 -> Gain2/1, Gain1/1
  Subsystem1/1(v) -> Mux1/1
  Subsystem2/1(v) -> Mux1/2
  Constant/1 -> Subsystem1/1(iref)
  Km/1 -> Subsystem2/4(Km)

== system MCU_regionalPolePlacementLMI_SAME54_MCLV2/Control/Electrical Control/Filter ==
  Input : Inport
  Delay11 : Delay  DelayLength=1  InitialCondition=0
  SumA21 : Sum  Inputs=|+-  RndMeth=Nearest  SaturateOnIntegerOverflow=on  OutDataTypeStr=Inherit: Same as first input
  SumB21 : Sum  Inputs=|++  RndMeth=Nearest  SaturateOnIntegerOverflow=on  OutDataTypeStr=Inherit: Same as first input
  a(2)(1) : Gain  Gain=-0.999371878778719136  ParamDataTypeStr=double  RndMeth=Nearest  SaturateOnIntegerOverflow=on  OutDataTypeStr=Inherit: Same as input
  s(1) : Gain  Gain=0.000314060610640442357  ParamDataTypeStr=double  RndMeth=Nearest  SaturateOnIntegerOverflow=on  OutDataTypeStr=Inherit: Same as input
  Output : Outport
  wires:
  Input/1 -> s(1)/1
  s(1)/1 -> SumA21/1
  SumA21/1 -> SumB21/1, Delay11/1
  SumB21/1 -> Output/1
  a(2)(1)/1 -> SumA21/2
  Delay11/1 -> a(2)(1)/1, SumB21/2

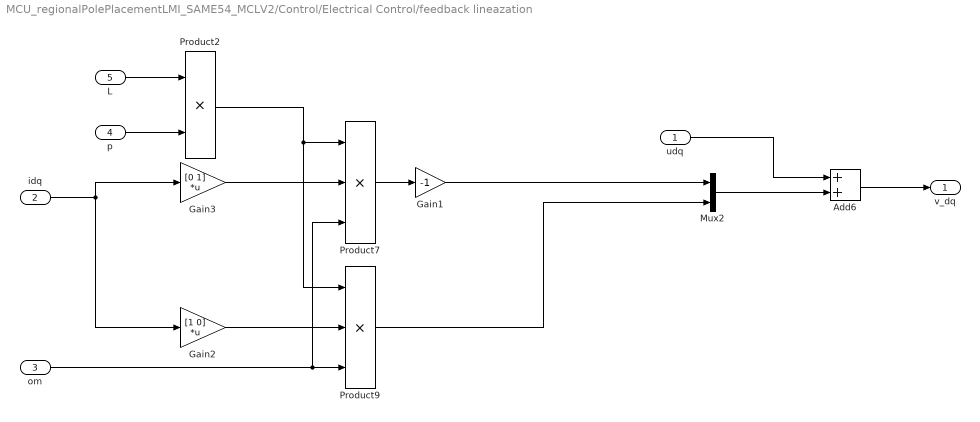
== system MCU_regionalPolePlacementLMI_SAME54_MCLV2/Control/Electrical Control/feedback lineazation ==
  udq : Inport
  idq : Inport  Port=2
  om : Inport  Port=3
  p : Inport  Port=4
  L : Inport  Port=5
  Add6 : Sum
  Gain1 : Gain  Gain=-1
  Gain2 : Gain  Gain=[1 0]  Multiplication=Matrix(K*u)
  Gain3 : Gain  Gain=[0 1]  Multiplication=Matrix(K*u)
  Mux2 : Mux  Inputs=2
  Product2 : Product
  Product7 : Product  Inputs=3
  Product9 : Product  Inputs=3
  v_dq : Outport  VectorParamsAs1DForOutWhenUnconnected=off
  wires:
  Mux2/1 -> Add6/2
  Product9/1 -> Mux2/2
  udq/1 -> Add6/1
  Add6/1 -> v_dq/1
  idq/1 -> Gain2/1, Gain3/1
  Gain1/1 -> Mux2/1
  p/1 -> Product2/2
  L/1 -> Product2/1
  Product2/1 -> Product9/1, Product7/1
  Gain3/1 -> Product7/2
  Product7/1 -> Gain1/1
  om/1 -> Product7/3, Product9/3
  Gain2/1 -> Product9/2

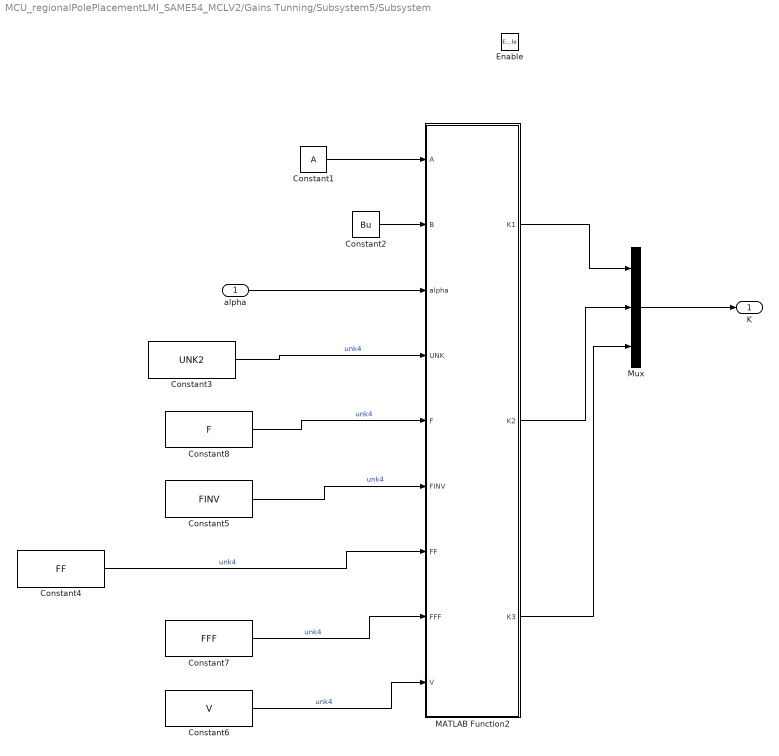
== system MCU_regionalPolePlacementLMI_SAME54_MCLV2/Gains Tunning/Subsystem5/Subsystem ==
  alpha : Inport
  Enable : EnablePort  StatesWhenEnabling=reset
  Constant1 : Constant  Value=A  OutDataTypeStr=single
  Constant2 : Constant  Value=Bu  OutDataTypeStr=single
  Constant3 : Constant  Value=UNK2  OutDataTypeStr=Bus: UNK_bus
  Constant4 : Constant  Value=FF  OutDataTypeStr=Bus: FF_bus
  Constant5 : Constant  Value=FINV  OutDataTypeStr=Bus: F_bus
  Constant6 : Constant  Value=V  OutDataTypeStr=Bus: FFF_bus
  Constant7 : Constant  Value=FFF  OutDataTypeStr=Bus: FFF_bus
  Constant8 : Constant  Value=F  OutDataTypeStr=Bus: F_bus
  MATLAB Function2 : MATLAB Function  TreatAsAtomicUnit=on
  Mux : Mux  Inputs=3
  K : Outport
  wires:
  Constant1/1 -> MATLAB Function2/1(A)
  Constant2/1 -> MATLAB Function2/2(B)
  alpha/1 -> MATLAB Function2/3(alpha)
  Mux/1 -> K/1
  MATLAB Function2/3(K3) -> Mux/3
  MATLAB Function2/2(K2) -> Mux/2
  MATLAB Function2/1(K1) -> Mux/1
  Constant8/1 -> MATLAB Function2/5(F)  "unk4"
  Constant5/1 -> MATLAB Function2/6(FINV)  "unk4"
  Constant3/1 -> MATLAB Function2/4(UNK)  "unk4"
  Constant7/1 -> MATLAB Function2/8(FFF)  "unk4"
  Constant6/1 -> MATLAB Function2/9(V)  "unk4"
  Constant4/1 -> MATLAB Function2/7(FF)  "unk4"

== system MCU_regionalPolePlacementLMI_SAME54_MCLV2/Gains Tunning/Subsystem5/Subsystem1 ==
  alpha : Inport
  Enable : EnablePort
  Constant : Constant  OutDataTypeStr=boolean
  Data Store Write : DataStoreWrite  DataStoreName=enable  IndexOptions=Index vector (dialog)  Indices=1  OutputSizes=1
  Data Store Write1 : DataStoreWrite  DataStoreName=alpha  IndexOptions=Index vector (dialog)  Indices=1  OutputSizes=1
  wires:
  alpha/1 -> Data Store Write1/1
  Constant/1 -> Data Store Write/1

== system MCU_regionalPolePlacementLMI_SAME54_MCLV2/Gains Tunning/Subsystem5/Subsystem2 ==
  Trigger : TriggerPort  VariantControl=(inherit)  PortDimensions=1
  Constant : Constant  Value=0  OutDataTypeStr=boolean
  Data Store Write : DataStoreWrite  DataStoreName=enable  IndexOptions=Index vector (dialog)  Indices=1  OutputSizes=1
  wires:
  Constant/1 -> Data Store Write/1

== system MCU_regionalPolePlacementLMI_SAME54_MCLV2/Motor Interface/Init Enc/Wait 1s ==
  AND : Logic  IconShape=distinctive  AllPortsSameDT=off  OutDataTypeStr=boolean
  Compare To Constant : simulink/Logic and Bit Operations/Compare To Constant  relop=>  const=1  OutDataTypeStr=boolean
  Compare To Constant1 : simulink/Logic and Bit Operations/Compare To Constant  relop=>  const=1.1  OutDataTypeStr=boolean
  Constant1 : Constant  OutDataTypeStr=int16
  Discrete-Time Integrator : DiscreteIntegrator  SampleTime=-1  SaturateOnIntegerOverflow=on  LimitOutput=on  UpperSaturationLimit=2  LowerSaturationLimit=0  ICPrevOutput=DiscIntNeverNeededParam  ICPrevScaledInput=DiscIntNeverNeededParam
  NOT : Logic  Operator=NOT  IconShape=distinctive  AllPortsSameDT=off  OutDataTypeStr=boolean
  init enc : Outport
  init done : Outport  Port=2
  wires:
  NOT/1 -> AND/2
  AND/1 -> init enc/1
  Compare To Constant1/1 -> NOT/1, init done/1
  Discrete-Time Integrator/1 -> Compare To Constant/1, Compare To Constant1/1
  Constant1/1 -> Discrete-Time Integrator/1
  Compare To Constant/1 -> AND/1

== system MCU_regionalPolePlacementLMI_SAME54_MCLV2/Control/Electrical Control/Current/Subsystem1 ==
  iref : Inport
  i : Inport  Port=2
  K_e : Inport  Port=3
  Discrete-Time Integrator : DiscreteIntegrator  SampleTime=-1  ICPrevOutput=DiscIntNeverNeededParam  ICPrevScaledInput=DiscIntNeverNeededParam
  Gain : Gain  Gain=[0 1]  Multiplication=Matrix(K*u)
  Gain1 : Gain  Gain=[1 0]  Multiplication=Matrix(K*u)
  Product : Product  OutDataTypeStr=single
  Product1 : Product  OutDataTypeStr=single
  Sum : Sum  Inputs=|--  OutDataTypeStr=single  SaturateOnIntegerOverflow=on
  Sum3 : Sum  Inputs=|+-
  v : Outport  VectorParamsAs1DForOutWhenUnconnected=off
  wires:
  Gain1/1 -> Product1/2
  Gain/1 -> Product/2
  K_e/1 -> Gain1/1, Gain/1
  Product1/1 -> Sum/2
  Product/1 -> Sum/1
  i/1 -> Product1/1, Sum3/2
  Sum3/1 -> Discrete-Time Integrator/1
  iref/1 -> Sum3/1
  Discrete-Time Integrator/1 -> Product/1
  Sum/1 -> v/1

== system MCU_regionalPolePlacementLMI_SAME54_MCLV2/Control/Electrical Control/Current/Subsystem2 ==
  omref : Inport
  om : Inport  Port=2
  i : Inport  Port=3
  Km : Inport  Port=4
  Add : Sum  Inputs=+++
  Demux : Demux  Outputs=3
  Discrete-Time Integrator : DiscreteIntegrator  SampleTime=-1  ICPrevOutput=DiscIntNeverNeededParam  ICPrevScaledInput=DiscIntNeverNeededParam
  Product : Product
  Product1 : Product
  Product2 : Product
  Sum3 : Sum  Inputs=|+-
  v : Outport  VectorParamsAs1DForOutWhenUnconnected=off
  wires:
  Add/1 -> v/1
  i/1 -> Product/1
  Sum3/1 -> Product2/1
  omref/1 -> Sum3/1
  om/1 -> Sum3/2, Product1/1
  Km/1 -> Demux/1
  Product2/1 -> Discrete-Time Integrator/1
  Product1/1 -> Add/2
  Product/1 -> Add/1
  Demux/1 -> Product/2
  Demux/2 -> Product1/2
  Demux/3 -> Product2/2
  Discrete-Time Integrator/1 -> Add/3
